simulink subsystem "control_alloc"  (R2025b)
settings: Solver=VariableStepAuto  StartTime=0.0  StopTime=10.0  RelTol=1e-3
values from neighbouring files (symbols this model uses):
  a = 13.06    [params.m]    (also in params_3dof.m = 13; test.m = 0.0013)
  b = 0.0859    [params.m]    (also in params_3dof.m = 0.085908; test.m = 8.5908)
settings Model: Creator=schwmaxi  LastModifiedBy=schwmaxi

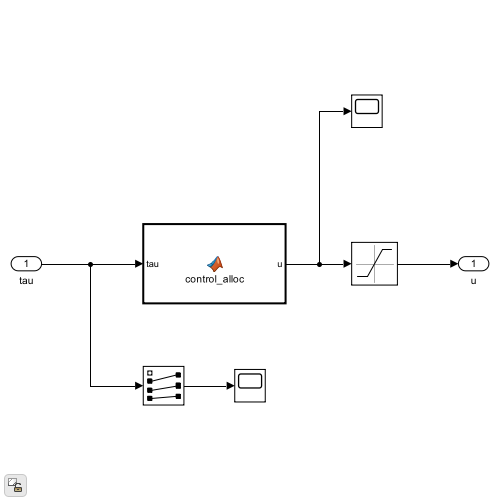
[thumbnail: Simulink's stored preview of the top-level diagram]
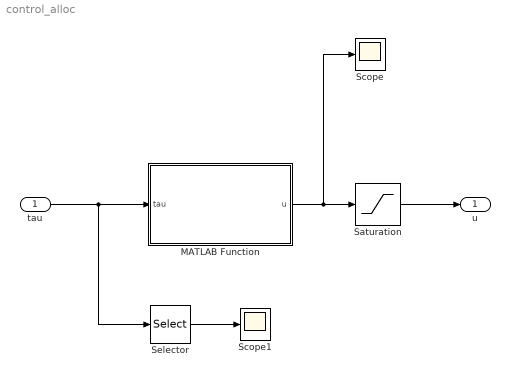
== system control_alloc ==
  tau : Inport
  MATLAB Function : MATLAB Function  TreatAsAtomicUnit=on
  Saturation : Saturate  UpperLimit=0.90  LowerLimit=0.15
  Scope : Scope
      settings: ActiveDisplayYMinimum=-27.935651021251019  ActiveDisplayYMaximum=101.5794361861844  DataLoggingVariableName=ScopeData2
  Scope1 : Scope
      settings: ActiveDisplayYMinimum=-0.010558305316975979  ActiveDisplayYMaximum=0.027496130370215789  DataLoggingVariableName=ScopeData3
  Selector : Selector  InputPortWidth=4  IndexOptions=Index vector (dialog)  Indices=[2 3 4]  OutputSizes=1
  u : Outport
  wires:
  Selector/1 -> Scope1/1
  Saturation/1 -> u/1
  tau/1 -> MATLAB Function/1(tau), Selector/1
  MATLAB Function/1(u) -> Scope/1, Saturation/1

== matlab function control_alloc/MATLAB Function ==
  data: tau input; u output; a parameter; b parameter; E parameter
function u = control_alloc(tau, a, b, E)
    % a, b, E werden als Parameter Data übergeben, vgl. Symbols Pane

    u = thrust_to_throttle(E \ tau, a, b);
end

function throttle = thrust_to_throttle(thrust, a, b)
    throttle = zeros(size(thrust));

    idx = thrust ./ a >= 0;
    throttle(idx) = sqrt(thrust(idx) ./ a) + b;
end
